simulink model "dcMotor"  (R2021a)
settings: Solver=VariableStepAuto  StartTime=0.0  StopTime=30  RelTol=1e-3
values from neighbouring files (symbols this model uses):
  J_ADAPTIVE = beta_hat(1)    [assignment5.m]
  J_LS = beta_hat(1)    [assignment5.m]
  J_RLS = beta_hat(1)    [assignment5.m]
  k_ADAPTIVE = 1/beta_hat(2)    [assignment5.m]
  k_LS = 1/beta_hat(2)    [assignment5.m]
  k_RLS = 1/beta_hat(2)    [assignment5.m]
libraries: simulink x2
settings Model: Creator=fabio  LastModifiedBy=fabio

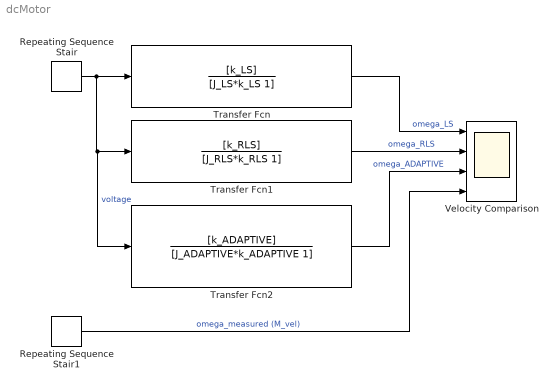
== system dcMotor ==
  Repeating Sequence Stair : simulink/Sources/Repeating Sequence Stair  OutValues=Y  tsamp=Ts  OutMin=[]  OutMax=[]  OutDataTypeStr=double  OutputDataTypeScalingMode=double  OutDataType=fixdt(0,8)  ConRadixGroup=Best Precision: Vector-wise  OutScaling=2^-12
  Repeating Sequence Stair1 : simulink/Sources/Repeating Sequence Stair  OutValues=M_vel  tsamp=Ts  OutMin=[]  OutMax=[]  OutDataTypeStr=double  OutputDataTypeScalingMode=double  OutDataType=fixdt(0,8)  ConRadixGroup=Best Precision: Vector-wise  OutScaling=2^-12
  Transfer Fcn : TransferFcn  Numerator=[k_LS]  Denominator=[J_LS*k_LS 1]
  Transfer Fcn1 : TransferFcn  Numerator=[k_RLS]  Denominator=[J_RLS*k_RLS 1]
  Transfer Fcn2 : TransferFcn  Numerator=[k_ADAPTIVE]  Denominator=[J_ADAPTIVE*k_ADAPTIVE 1]
  Velocity Comparison : Scope  NumInputPorts=4
  wires:
  Transfer Fcn/1 -> Velocity Comparison/1  "omega_LS"
  Repeating Sequence Stair/1 -> Transfer Fcn2/1, Transfer Fcn1/1, Transfer Fcn/1  "voltage"
  Transfer Fcn1/1 -> Velocity Comparison/2  "omega_RLS"
  Transfer Fcn2/1 -> Velocity Comparison/3  "omega_ADAPTIVE"
  Repeating Sequence Stair1/1 -> Velocity Comparison/4  "omega_measured (M_vel)"
